simulink subsystem "MCD"  (R2022b)
settings: Solver=VariableStepAuto  StartTime=0.0  StopTime=10.0  RelTol=1e-3
undefined symbols (not defined in the file): d
settings Model: Creator=David  LastModifiedBy=dar.io

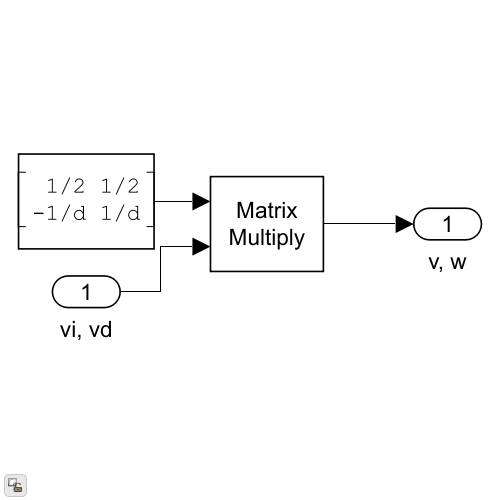
[thumbnail: Simulink's stored preview of the top-level diagram]
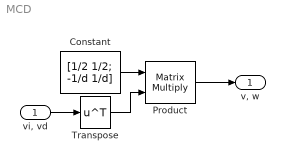
== system MCD ==
  "vi, vd" : Inport
  Constant : Constant  Value=[1/2 1/2; -1/d 1/d]
  Product : Product  Multiplication=Matrix(*)
  Transpose : Math  Operator=transpose
  "v, w" : Outport
  wires:
  Product/1 -> "v, w"/1
  Constant/1 -> Product/1
  "vi, vd"/1 -> Transpose/1
  Transpose/1 -> Product/2
